simulink library "Generator_Lib"  (R2014a)
settings: Solver=ode45  StartTime=0.0  StopTime=10.0  RelTol=1e-3
undefined symbols (not defined in the file): block_angle, D1, Delta, DiscIntNeverNeededParam, fao, gcbh, sps_rtmsupport, Ts
libraries: powerlib x73, simulink x16, powerlib_extras x13, Generator_Lib x3, sps_avr x2, powerlib_meascontrol x2, spsSimpleSynchronousMachineModel x2
(part 1 of 3)
Description:
  | Copyright 2014 The MathWorks, Inc.
settings Model: Creator=smiller  LastModifiedBy=psanghvi

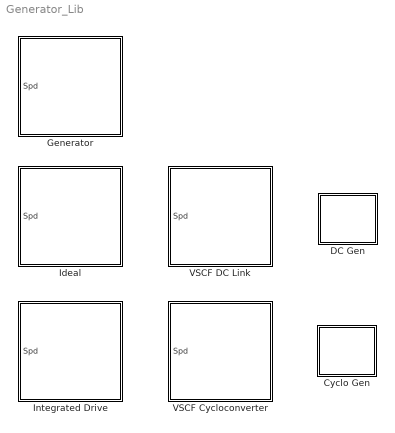
== system Generator_Lib ==
  Cyclo Gen : Subsystem
  DC Gen : Subsystem
  Generator : Subsystem  BlockChoice=Integrated Drive
      settings: TemplateBlock=self  MemberBlocks=Ideal,Integrated Drive,VSCF Cycloconverter,VSCF DC Link
  Ideal : Subsystem
      mask Display:
      | image(imread('Gen_Ideal_IMAGE.JPG','jpg'))
      | %port_label('RConn',1,'A');
      | %port_label('RConn',2,'B');
      | %port_label('RConn',3,'C');
      | %port_label('Input',1,'Spd');
  Integrated Drive : Subsystem
      mask Display:
      | image(imread('Gen_IDG_IMAGE.JPG','jpg'))
      | %port_label('RConn',1,'A');
      | %port_label('RConn',2,'B');
      | %port_label('RConn',3,'C');
      | %port_label('Input',1,'Spd');
  VSCF Cycloconverter : Subsystem
      mask Display:
      | image(imread('Gen_VSCF_Cycloconverter_IMAGE.JPG','jpg'))
      | %port_label('RConn',1,'A');
      | %port_label('RConn',2,'B');
      | %port_label('RConn',3,'C');
      | %port_label('Input',1,'Spd');
  VSCF DC Link : Subsystem
      mask Display:
      | image(imread('Gen_VSCF_DCLink_IMAGE.JPG','jpg'))
      | %port_label('RConn',1,'A');
      | %port_label('RConn',2,'B');
      | %port_label('RConn',3,'C');
      | %port_label('Input',1,'Spd');

== system Generator_Lib/Cyclo Gen ==
  Ideal : Subsystem
      mask Display:
      | image(imread('Gen_Ideal_Var_IMAGE.jpg'));
      | port_label('RConn',1,'A');
      | port_label('RConn',2,'B');
      | port_label('RConn',3,'C');
      | port_label('Input',1,'rpm');

== system Generator_Lib/DC Gen ==
  DC Link Gen : Subsystem  BlockChoice=Ideal
      settings: TemplateBlock=self  MemberBlocks=Ideal,Sync Mach
  Ideal : Subsystem
      mask Display: image(imread('Gen_Ideal_Var_IMAGE.jpg'));
  Sync Mach : Subsystem
      mask Display: image(imread('Gen_Sync_Machine_IMAGE.jpg'));

== system Generator_Lib/Generator ==
  Spd : Inport
  Integrated Drive : Generator_Lib/Integrated Drive  SystemSampleTime=-1
  A : PMIOPort  Port=1  Side=Right
  B : PMIOPort  Port=2  Side=Right
  C : PMIOPort  Port=3  Side=Right
  wires:
  Spd/1 -> Integrated Drive/1
  connections:
  Integrated Drive/RConn1 -- A/RConn1
  Integrated Drive/RConn2 -- B/RConn1
  Integrated Drive/RConn3 -- C/RConn1

== system Generator_Lib/Ideal ==
  Spd : Inport
  Parasitic Resistive Load : powerlib/Elements/Three-Phase Series RLC Load  LConnTagsString=A|B|C  Configuration=Y (grounded)  NominalVoltage=200  NominalFrequency=400  ActivePower=5000  InductivePower=0  CapacitivePower=0  Measurements=None  LoadType=constant Z
  Sensing : Subsystem
      mask Display: disp('S')
  Terminator : Terminator
  Three-Phase V-I Measurement4 : powerlib/Measurements/Three-Phase V-I Measurement  VoltageMeasurement=phase-to-ground  SetLabelV=on  LabelV=Vabc_Gen1Only  Vpu=off  VpuLL=off  CurrentMeasurement=yes  SetLabelI=on  LabelI=Iabc_Gen1Only  Ipu=off  Pbase=100e6  Vbase=500e3  OutputType=Magnitude  PhasorSimulation=on  PSBequivalent=0
  Three-Phase Source : powerlib/Electrical Sources/Three-Phase Source  Voltage=200  PhaseAngle=0  Frequency=400  InternalConnection=Yg  SpecifyImpedance=off  Resistance=0.1*0  Inductance=0.01*0  ShortCircuitLevel=0.1  BaseVoltage=200  XRratio=7  BusType=swing  Pref=0  Qref=0  Qmin=-inf  Qmax=inf
  Vab : Subsystem
  rpm2 radps : Gain  Gain=pi/30
  A : PMIOPort  Port=1  Side=Right
  B : PMIOPort  Port=2  Side=Right
  C : PMIOPort  Port=3  Side=Right
  wires:
  Spd/1 -> rpm2 radps/1
  rpm2 radps/1 -> Terminator/1
  connections:
  Vab/RConn2 -- Three-Phase V-I Measurement4/RConn2 -- Parasitic Resistive Load/LConn2 -- B/RConn1
  Parasitic Resistive Load/LConn3 -- Three-Phase V-I Measurement4/RConn3 -- C/RConn1
  Vab/RConn1 -- Three-Phase V-I Measurement4/RConn1 -- Parasitic Resistive Load/LConn1 -- A/RConn1
  Three-Phase V-I Measurement4/LConn1 -- Three-Phase Source/RConn1
  Three-Phase V-I Measurement4/LConn2 -- Three-Phase Source/RConn2
  Three-Phase V-I Measurement4/LConn3 -- Three-Phase Source/RConn3

== system Generator_Lib/Integrated Drive ==
  Spd : Inport
  Bus Selector2 : BusSelector  OutputSignals=Rotor speed wm (rad/s)
  Displays : Subsystem
  Generator Control Unit (GCU) : Subsystem
      mask Display: %image(imread('power_aircraft_distribution_GCU.jpg','jpg'))
  Generator Control Breaker (GCB) : Subsystem
  IDG : Subsystem
  Parasitic Resistive Load : powerlib/Elements/Three-Phase Series RLC Load  LConnTagsString=A|B|C  Configuration=Y (grounded)  NominalVoltage=200  NominalFrequency=400  ActivePower=5000  InductivePower=0  CapacitivePower=0  Measurements=None  LoadType=constant Z
  Sensing : Subsystem
      mask Display: disp('S')
  Simplified Synchronous Machine SI Units : powerlib/Machines/Simplified Synchronous Machine SI Units  ConnectionType=3-wire Y  MechanicalLoad=Speed w  MeasurementBus=off  NominalParameters=[50e3 200 400]  Mechanical=[0.02 0 2]  InternalRL="[0.0204  0.08104e-3]"  InitialConditions=[-99 1.73677 24.5109 24.5109 24.5109 -1.98949 -121.989 118.011]  Units=1  LoadFlowParameters=[1 0 0 0 0]  TsPowergui=0  TsBlock=-1  BusType=swing  Pref=0  Qref=0  Qmin=-inf  Qmax=+inf  PLF=0  QLF=0
  Vab : Subsystem
  A : PMIOPort  Port=1  Side=Right
  B : PMIOPort  Port=2  Side=Right
  C : PMIOPort  Port=3  Side=Right
  wires:
  Simplified Synchronous Machine SI Units/1 -> Sensing/1(In1), Bus Selector2/1
  Generator Control Breaker (GCB)/1(Vabc) -> Generator Control Unit (GCU)/2(Vabc)
  Bus Selector2/1 -> Generator Control Breaker (GCB)/1(GLC), Generator Control Unit (GCU)/3(PMG), Displays/1(w)  "<Rotor speed wm (rad/s)>"
  Generator Control Unit (GCU)/1(V Field) -> Simplified Synchronous Machine SI Units/2  "Field"
  Generator Control Breaker (GCB)/2(Iabc) -> Generator Control Unit (GCU)/1(Iabc)
  Spd/1 -> IDG/1(Tur)
  IDG/1(Dr) -> Simplified Synchronous Machine SI Units/1
  connections:
  A/RConn1 -- Vab/RConn1 -- Generator Control Breaker (GCB)/RConn1
  C/RConn1 -- Generator Control Breaker (GCB)/RConn3
  B/RConn1 -- Vab/RConn2 -- Generator Control Breaker (GCB)/RConn2
  Generator Control Breaker (GCB)/LConn3 -- Parasitic Resistive Load/LConn3 -- Simplified Synchronous Machine SI Units/RConn3
  Parasitic Resistive Load/LConn2 -- Generator Control Breaker (GCB)/LConn2 -- Simplified Synchronous Machine SI Units/RConn2
  Parasitic Resistive Load/LConn1 -- Generator Control Breaker (GCB)/LConn1 -- Simplified Synchronous Machine SI Units/RConn1

== system Generator_Lib/VSCF Cycloconverter ==
  Spd : Inport
  AC Generator Cycloconverter : Subsystem
  Constant : Constant  Value=[0 0 0]
  Generator Control Breaker (GCB) : Subsystem
  Terminator : Terminator
  Terminator1 : Terminator
  Vab : Subsystem
  A : PMIOPort  Port=1  Side=Right
  B : PMIOPort  Port=2  Side=Right
  C : PMIOPort  Port=3  Side=Right
  tag scope: Gen1Bus=global
  wires:
  Spd/1 -> AC Generator Cycloconverter/1(rpm), Generator Control Breaker (GCB)/1(GLC)
  Constant/1 -> [Gen1Bus]
  Generator Control Breaker (GCB)/1(Vabc) -> Terminator/1
  Generator Control Breaker (GCB)/2(Iabc) -> Terminator1/1
  connections:
  Vab/RConn1 -- Generator Control Breaker (GCB)/RConn1 -- A/RConn1
  C/RConn1 -- Generator Control Breaker (GCB)/RConn3
  Vab/RConn2 -- Generator Control Breaker (GCB)/RConn2 -- B/RConn1
  AC Generator Cycloconverter/RConn3 -- Generator Control Breaker (GCB)/LConn3
  AC Generator Cycloconverter/RConn2 -- Generator Control Breaker (GCB)/LConn2
  AC Generator Cycloconverter/RConn1 -- Generator Control Breaker (GCB)/LConn1

== system Generator_Lib/VSCF DC Link ==
  note: AC-DC-AC PWM Converter
  Spd : Inport
  Constant : Constant  Value=[0 0 0]
  DC Link Gen : Subsystem  BlockChoice=Ideal
      settings: AttributesFormatString=%<BlockChoice>  TemplateBlock=Generator_Lib/DC Gen/DC Link Gen  MemberBlocks=Ideal,Sync Mach
  LC Filter : Subsystem
  Meas : powerlib/Measurements/Three-Phase V-I Measurement  VoltageMeasurement=phase-to-ground  SetLabelV=off  LabelV=V1  Vpu=on  VpuLL=off  CurrentMeasurement=no  SetLabelI=off  LabelI=I1  Ipu=off  Pbase=1e3  Vbase=200  OutputType=Magnitude  PhasorSimulation=off  PSBequivalent=0
  Rect and Inv : Subsystem
  Regulator : Subsystem
  Subsystem2 : Subsystem
      mask Display: disp('S')
  Subsystem4 : Subsystem
      mask Display: disp('S')
  Subsystem5 : Subsystem
      mask Display: disp('S')
  Transformer : powerlib/Elements/Three-Phase Transformer (Two Windings)  Winding1Connection=Yg  UNITS=pu  NominalPower=[ 50e3 , 800 ]  Winding1=[ 200 , 0.004 , 0.02 ]  Winding2Connection=Delta (D1)  Winding2=[ 600 , 0.004 , 0.02 ]  SetSaturation=off  Rm=200  Lm=200  Saturation="[ 0,0  ;  0.005,1.2  ;  1.0,1.4 ]"  Hysteresis=off  DataFile='hysteresis'  SetInitialFlux=off  InitialFluxes=[ 0.8 , -0.8 , 0.7 ]  Measurements=None  MoreParameters=off  BreakLoop=off  DataType=off  TransfoNumber=0
  "Vref (pu) " : Constant
  A : PMIOPort  Port=1  Side=Right
  B : PMIOPort  Port=2  Side=Right
  C : PMIOPort  Port=3  Side=Right
  tag scope: Gen1Bus=global
  wires:
  "Vref (pu) "/1 -> Regulator/1(Vref (pu))
  Meas/1 -> Regulator/2(Vabc (pu))
  Regulator/1(g) -> Rect and Inv/1(g)
  Spd/1 -> DC Link Gen/1(rpm)
  Constant/1 -> [Gen1Bus]
  connections:
  Subsystem4/LConn1 -- A/RConn1 -- Meas/RConn1
  Transformer/LConn1 -- DC Link Gen/RConn1 -- Subsystem2/LConn1
  LC Filter/LConn2 -- Rect and Inv/RConn2 -- Subsystem5/LConn2
  LC Filter/LConn1 -- Subsystem5/LConn1 -- Rect and Inv/RConn1
  B/RConn1 -- Meas/RConn2
  Meas/LConn1 -- LC Filter/RConn1
  DC Link Gen/RConn2 -- Transformer/LConn2
  Meas/LConn2 -- LC Filter/RConn2
  Meas/RConn3 -- C/RConn1
  Meas/LConn3 -- LC Filter/RConn3
  Transformer/RConn1 -- Rect and Inv/LConn1
  DC Link Gen/RConn3 -- Transformer/LConn3
  Rect and Inv/LConn2 -- Transformer/RConn2
  Transformer/RConn3 -- Rect and Inv/LConn3
  Rect and Inv/RConn3 -- LC Filter/LConn3

== system Generator_Lib/Cyclo Gen/Ideal ==
  rpm : Inport
  Cycloconverter control (Vsync) : Subsystem
  Ground1 : powerlib/Elements/Ground  LConnTagsString=a
  Ideal Source : Subsystem
  Load Measurements : powerlib/Measurements/Three-Phase V-I Measurement  VoltageMeasurement=phase-to-ground  SetLabelV=on  LabelV=Vload  Vpu=off  VpuLL=off  CurrentMeasurement=yes  SetLabelI=on  LabelI=Iload  Ipu=off  Pbase=100e6  Vbase=500e3  OutputType=Complex  PhasorSimulation=off  PSBequivalent=0
  Phase A Cycloconverter : Subsystem
  Phase B Cycloconverter : Subsystem
  Phase C Cycloconverter : Subsystem
  Source Measurements : powerlib/Measurements/Three-Phase V-I Measurement  VoltageMeasurement=phase-to-ground  SetLabelV=on  LabelV=Vsource  Vpu=off  VpuLL=off  CurrentMeasurement=yes  SetLabelI=on  LabelI=Isource  Ipu=off  Pbase=100e6  Vbase=500e3  OutputType=Complex  PhasorSimulation=off  PSBequivalent=0
  Three-Phase Transformer (Two Windings)1 : powerlib/Elements/Three-Phase Transformer (Two Windings)  Winding1Connection=Delta (D1)  UNITS=pu  NominalPower=[3e6 3000]  Winding1=[200 0 0]  Winding2Connection=Delta (D1)  Winding2=[200/sqrt(3) 1e-8 0]  SetSaturation=off  Rm=Inf  Lm=Inf  Saturation=[ 0,0 ; 0.0024,1.2 ; 1.0,1.52 ]  Hysteresis=off  DataFile='hysteresis'  SetInitialFlux=off  InitialFluxes=[ 0.8 , -0.8 , 0.7 ]  Measurements=None  MoreParameters=off  BreakLoop=off  DataType=off  TransfoNumber=1
  Three-Phase Transformer (Two Windings)2 : powerlib/Elements/Three-Phase Transformer (Two Windings)  Winding1Connection=Delta (D1)  UNITS=pu  NominalPower=[3e6 3000]  Winding1=[200 0 0]  Winding2Connection=Delta (D1)  Winding2=[200/sqrt(3) 1e-8 0]  SetSaturation=off  Rm=Inf  Lm=Inf  Saturation=[ 0,0 ; 0.0024,1.2 ; 1.0,1.52 ]  Hysteresis=off  DataFile='hysteresis'  SetInitialFlux=off  InitialFluxes=[ 0.8 , -0.8 , 0.7 ]  Measurements=None  MoreParameters=off  BreakLoop=off  DataType=off  TransfoNumber=1
  Three-Phase Transformer (Two Windings)3 : powerlib/Elements/Three-Phase Transformer (Two Windings)  Winding1Connection=Delta (D1)  UNITS=pu  NominalPower=[3e6 3000]  Winding1=[200 0 0]  Winding2Connection=Delta (D1)  Winding2=[200/sqrt(3) 1e-8 0]  SetSaturation=off  Rm=Inf  Lm=Inf  Saturation=[ 0,0 ; 0.0024,1.2 ; 1.0,1.52 ]  Hysteresis=off  DataFile='hysteresis'  SetInitialFlux=off  InitialFluxes=[ 0.8 , -0.8 , 0.7 ]  Measurements=None  MoreParameters=off  BreakLoop=off  DataType=off  TransfoNumber=1
  Vsync Measurement : powerlib/Measurements/Three-Phase V-I Measurement  VoltageMeasurement=phase-to-phase  SetLabelV=on  LabelV=Vsync  Vpu=off  VpuLL=off  CurrentMeasurement=no  SetLabelI=off  LabelI=Iabc  Ipu=off  Pbase=100e6  Vbase=500e3  OutputType=Complex  PhasorSimulation=off  PSBequivalent=0
  A : PMIOPort  Port=1  Side=Right
  B : PMIOPort  Port=2  Side=Right
  C : PMIOPort  Port=3  Side=Right
  wires:
  rpm/1 -> Ideal Source/1(rpm)
  connections:
  Load Measurements/RConn1 -- A/RConn1
  Phase A Cycloconverter/LConn2 -- Vsync Measurement/RConn2
  Three-Phase Transformer (Two Windings)3/RConn3 -- Vsync Measurement/LConn3
  Phase C Cycloconverter/RConn2 -- Phase A Cycloconverter/RConn2 -- Phase B Cycloconverter/RConn2 -- Ground1/LConn1
  Three-Phase Transformer (Two Windings)2/RConn2 -- Phase C Cycloconverter/LConn2
  Source Measurements/RConn3 -- Three-Phase Transformer (Two Windings)3/LConn3 -- Three-Phase Transformer (Two Windings)2/LConn3 -- Three-Phase Transformer (Two Windings)1/LConn3
  Phase B Cycloconverter/RConn1 -- Load Measurements/LConn2
  Vsync Measurement/RConn1 -- Phase A Cycloconverter/LConn1
  Phase B Cycloconverter/LConn1 -- Three-Phase Transformer (Two Windings)1/RConn1
  Phase B Cycloconverter/LConn2 -- Three-Phase Transformer (Two Windings)1/RConn2
  Three-Phase Transformer (Two Windings)3/RConn1 -- Vsync Measurement/LConn1
  Phase C Cycloconverter/LConn1 -- Three-Phase Transformer (Two Windings)2/RConn1
  Phase A Cycloconverter/RConn1 -- Load Measurements/LConn1
  Source Measurements/RConn1 -- Three-Phase Transformer (Two Windings)3/LConn1 -- Three-Phase Transformer (Two Windings)2/LConn1 -- Three-Phase Transformer (Two Windings)1/LConn1
  Source Measurements/RConn2 -- Three-Phase Transformer (Two Windings)3/LConn2 -- Three-Phase Transformer (Two Windings)2/LConn2 -- Three-Phase Transformer (Two Windings)1/LConn2
  Phase C Cycloconverter/RConn1 -- Load Measurements/LConn3
  Vsync Measurement/RConn3 -- Phase A Cycloconverter/LConn3
  Load Measurements/RConn3 -- C/RConn1
  Phase C Cycloconverter/LConn3 -- Three-Phase Transformer (Two Windings)2/RConn3
  Source Measurements/LConn2 -- Ideal Source/RConn2
  Three-Phase Transformer (Two Windings)3/RConn2 -- Vsync Measurement/LConn2
  Ideal Source/RConn1 -- Source Measurements/LConn1
  Load Measurements/RConn2 -- B/RConn1
  Ideal Source/RConn3 -- Source Measurements/LConn3
  Three-Phase Transformer (Two Windings)1/RConn3 -- Phase B Cycloconverter/LConn3

== system Generator_Lib/DC Gen/DC Link Gen ==
  rpm : Inport
  Ideal : Generator_Lib/DC Gen/Ideal  SystemSampleTime=-1
  A : PMIOPort  Port=1  Side=Right
  B : PMIOPort  Port=2  Side=Right
  C : PMIOPort  Port=3  Side=Right
  wires:
  rpm/1 -> Ideal/1
  connections:
  Ideal/RConn1 -- A/RConn1
  Ideal/RConn2 -- B/RConn1
  Ideal/RConn3 -- C/RConn1

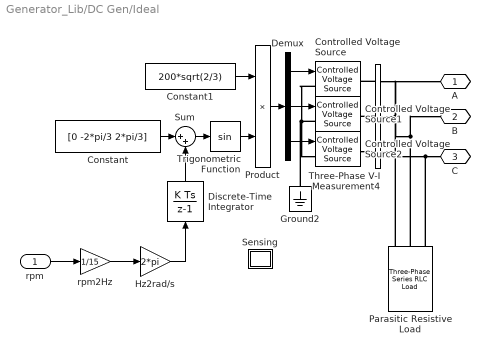
== system Generator_Lib/DC Gen/Ideal ==
  rpm : Inport
  Constant : Constant  Value=[0 -2*pi/3 2*pi/3]
  Constant1 : Constant  Value=200*sqrt(2/3)
  Controlled Voltage Source : powerlib/Electrical Sources/Controlled Voltage Source  Initialize=off  Source_Type=AC  Amplitude=0  Phase=0  Frequency=0  Measurements=None
  Controlled Voltage Source1 : powerlib/Electrical Sources/Controlled Voltage Source  Initialize=off  Source_Type=AC  Amplitude=0  Phase=0  Frequency=0  Measurements=None
  Controlled Voltage Source2 : powerlib/Electrical Sources/Controlled Voltage Source  Initialize=off  Source_Type=AC  Amplitude=0  Phase=0  Frequency=0  Measurements=None
  Demux : Demux  Outputs=3
  Discrete-Time Integrator : DiscreteIntegrator  SampleTime=Ts  ICPrevOutput=DiscIntNeverNeededParam  ICPrevScaledInput=DiscIntNeverNeededParam
  Ground2 : powerlib/Elements/Ground  LConnTagsString=a
  Hz2rad/s : Gain  Gain=2*pi
  Parasitic Resistive Load : powerlib/Elements/Three-Phase Series RLC Load  LConnTagsString=A|B|C  Configuration=Y (grounded)  NominalVoltage=200  NominalFrequency=400  ActivePower=5000  InductivePower=0  CapacitivePower=0  Measurements=None  LoadType=constant Z
  Product : Product
  Sensing : Subsystem
      mask Display: disp('S')
  Sum : Sum  Inputs=|++
  Three-Phase V-I Measurement4 : powerlib/Measurements/Three-Phase V-I Measurement  VoltageMeasurement=phase-to-ground  SetLabelV=on  LabelV=Vabc_Gen1Only  Vpu=off  VpuLL=off  CurrentMeasurement=yes  SetLabelI=on  LabelI=Iabc_Gen1Only  Ipu=off  Pbase=100e6  Vbase=500e3  OutputType=Magnitude  PhasorSimulation=on  PSBequivalent=0
  Trigonometric Function : Trigonometry
  rpm2Hz : Gain  Gain=1/15
  A : PMIOPort  Port=1  Side=Right
  B : PMIOPort  Port=2  Side=Right
  C : PMIOPort  Port=3  Side=Right
  wires:
  rpm/1 -> rpm2Hz/1
  Discrete-Time Integrator/1 -> Sum/2
  Constant1/1 -> Product/1
  Constant/1 -> Sum/1
  Hz2rad/s/1 -> Discrete-Time Integrator/1
  Sum/1 -> Trigonometric Function/1
  Trigonometric Function/1 -> Product/2
  Product/1 -> Demux/1
  Demux/1 -> Controlled Voltage Source/1
  Demux/2 -> Controlled Voltage Source1/1
  Demux/3 -> Controlled Voltage Source2/1
  rpm2Hz/1 -> Hz2rad/s/1
  connections:
  Controlled Voltage Source/LConn1 -- Ground2/LConn1 -- Controlled Voltage Source2/LConn1 -- Controlled Voltage Source1/LConn1
  Three-Phase V-I Measurement4/LConn1 -- Controlled Voltage Source/RConn1
  Three-Phase V-I Measurement4/LConn2 -- Controlled Voltage Source1/RConn1
  Controlled Voltage Source2/RConn1 -- Three-Phase V-I Measurement4/LConn3
  Three-Phase V-I Measurement4/RConn3 -- Parasitic Resistive Load/LConn3 -- C/RConn1
  Three-Phase V-I Measurement4/RConn2 -- Parasitic Resistive Load/LConn2 -- B/RConn1
  Three-Phase V-I Measurement4/RConn1 -- A/RConn1 -- Parasitic Resistive Load/LConn1

== system Generator_Lib/DC Gen/Sync Mach ==
  rpm : Inport
  Bus Selector2 : BusSelector  OutputSignals=Rotor speed wm (rad/s)
  Displays : Subsystem
  Generator Control Unit (GCU) : Subsystem
      mask Display: %image(imread('power_aircraft_distribution_GCU.jpg','jpg'))
  Generator Control Breaker (GCB) : Subsystem
  Parasitic Resistive Load : PMComponent  DialogController=POWERSYS.PowerSysDialog  LoadFcn=sps_rtmsupport('LoadFcn',gcbh);  StartFcn=sps_rtmsupport('StartFcn',gcbh);  StopFcn=sps_rtmsupport('StopFcn',gcbh);  PhysicalDomain=powersysdomain  LeftPortType=p1  RightPortType=p1  LConnTagsString=A|B|C  mask(Three-Phase Series RLC Load){Configuration=Y (grounded), NominalVoltage=200, NominalFrequency=800, ActivePower=5000, InductivePower=0, CapacitivePower=0, Measurements=None, LoadType=constant Z}
      mask prompts: NominalVoltage "Nominal phase-to-phase voltage Vn (Vrms)"; NominalFrequency "Nominal frequency fn (Hz):"; ActivePower "Active power P (W):"; InductivePower "Inductive reactive power QL (positive var):"; CapacitivePower "Capacitive reactive power Qc (negative var):"; LoadType "Load type"
      mask help: Implements a three-phase series RLC load.
      mask init:
      | [s1,s2,s3,s4,r1,r2,l1,l2,c1,c2,c3,c4] = powericon('Series RLC Load',ActivePower,InductivePower,CapacitivePower);
      | ground = Configuration==1;
      | neutral = Configuration==3;
      | power_initmask();
      settings: AttributesFormatString=\n  CopyFcn=sps_rtmsupport('CopyFcn',gcbh);  DeleteFcn=sps_rtmsupport('DeleteFcn',gcbh);  UndoDeleteFcn=sps_rtmsupport('UndoDeleteFcn',gcbh);  ModelCloseFcn=sps_rtmsupport('ModelCloseFcn',gcbh);  PreSaveFcn=sps_rtmsupport('PreSaveFcn',gcbh);  PostSaveFcn=sps_rtmsupport('PostSaveFcn',gcbh);  NameChangeFcn=sps_rtmsupport('NameChangeFcn',gcbh);  PreCopyFcn=sps_rtmsupport('PreCopyFcn',gcbh);  OpenFcn=sps_rtmsupport('OpenFcn',gcbh, [1 7 8]);  CloseFcn=sps_rtmsupport('CloseFcn',gcbh);  PreDeleteFcn=sps_rtmsupport('PreDeleteFcn',gcbh);
      mask Help: helpview(psbhelp);
      mask TypeOptions Configuration: Y (grounded) | Y (floating) | Y (neutral) | Delta
      mask Callback Configuration: powericon('psbcallbacks',gcb,'Three-Phase Series RLC Load');
      mask TypeOptions Measurements: None | Branch voltages | Branch currents | Branch voltages and currents
      mask TypeOptions LoadType: constant Z | constant PQ
      mask Display:
      | plot(s1-60,s2,s3+80,s4,r1,r2,l1,l2,c1,c2,c3,c4)
      | 
      | plot( ground*[s3,s3], ground*[-s2/4,s2/4])
      | plot( ground*[s3+30,s3+30], ground*[-s2/6,s2/6])
      | plot( ground*[s3+60,s3+60], ground*[-s2/10,s2/10])
      | 
      | plot( neutral*[s3,s3+80], neutral*[0,0])
      | 
      | port_label('LConn', 1, 'A')
      | port_label('LConn', 2, 'B')
      | port_label('LConn', 3, 'C')
  Sensing : Subsystem
      mask Display: disp('S')
  Simplified Synchronous Machine SI Units : Subsystem  DialogController=POWERSYS.PowerSysDialog  LoadFcn=sps_rtmsupport('LoadFcn',gcbh);  StartFcn=sps_rtmsupport('StartFcn',gcbh);  StopFcn=sps_rtmsupport('StopFcn',gcbh);  mask(Simplified Synchronous Machine){ConnectionType=3-wire Y, MechanicalLoad=Speed w, NominalParameters=[50e3 200 800], Mechanical=[0.02 0 2*2], InternalRL=[0.0204  0.08104e-3], InitialConditions=[-99 1.73677 24.5109 24.5109 24.5109 -1.98949 -121.989 118.011], Units=1, LoadFlowParameters=[1 0 0 0 0], TsPowergui=0, TsBlock=-1, BusType=swing, Pref=0, Qref=0, Qmin=-inf, Qmax=+inf, PLF=0, QLF=0}
      mask prompts: ConnectionType "Connection type:"; MechanicalLoad "Mechanical input:"; NominalParameters "Nominal power, line-to-line voltage, and frequency [ Pn(VA) Vn(Vrms) fn(Hz) ]:"; Mechanical "Inertia, damping factor and pairs of poles [J(kg.m^2) Kd(pu_T/pu_w) p()]"; InternalRL "Internal impedance [ R(ohm)  L(H) ]:"; InitialConditions "Initial conditions [ dw(%)  th(deg)  ia,ib,ic(A)  pha,phb,phc(deg) ]:"; Units "iounits"; LoadFlowParameters "Load Flow Parameters"; TsPowergui "Sample time of powergui block"; TsBlock "Sample time (-1 for inherited)"; BusType "Generation type"; Pref "Active power generation P (W)"; Qref "Reactive power generation Q (var)"; Qmin "Minimum reactive power Qmin (var)"; Qmax "Maximum reactive power Qmax (var)"; PLF "Load flow solution P_LF (W)"; QLF "Load flow solution Q_LF (var)"
      mask help:
      | Implements a 3-phase simplified synchronous machine. Machine is modelled as an internal voltage behind a R-L impedance. Stator windings are connected in wye to an internal neutral point.
      |
      | Use this block if you want to specify SI  parameters.
      mask init:
      | block = gcb;
      | [Ts,SSM,WantBlockChoice,X,Y] = powericon('SimplifiedSynchronousMachineInit',block,TsPowergui,TsBlock,MechanicalLoad,'SI',ConnectionType,NominalParameters,Mechanical,InternalRL,InitialConditions,0,-1);
      | powericon('SetInternalModels','set',block,WantBlockChoice);
      | powericon('ShaftInput',block);
      settings: CopyFcn=sps_rtmsupport('CopyFcn',gcbh); powericon('psbloadfunction',gcb,'gotofrom','UpdateGotoTag');  DeleteFcn=sps_rtmsupport('DeleteFcn',gcbh);  UndoDeleteFcn=sps_rtmsupport('UndoDeleteFcn',gcbh);  ModelCloseFcn=sps_rtmsupport('ModelCloseFcn',gcbh);  PreSaveFcn=sps_rtmsupport('PreSaveFcn',gcbh);  PostSaveFcn=sps_rtmsupport('PostSaveFcn',gcbh);  NameChangeFcn=sps_rtmsupport('NameChangeFcn',gcbh);  PreCopyFcn=sps_rtmsupport('PreCopyFcn',gcbh);  OpenFcn=sps_rtmsupport('OpenFcn',gcbh, [1 2 11]);  CloseFcn=sps_rtmsupport('CloseFcn',gcbh);  PreDeleteFcn=sps_rtmsupport('PreDeleteFcn',gcbh);
      mask Help: helpview(psbhelp);
      mask TypeOptions ConnectionType: 3-wire Y | 4-wire Y
      mask Callback ConnectionType: powericon('SimplifiedSynchronousMachineCback',gcb);
      mask TypeOptions MechanicalLoad: Mechanical power Pm | Speed w | Mechanical rotational port
      mask TypeOptions BusType: swing | PV | PQ
      mask Callback BusType: powericon('SimplifiedSynchronousMachineCback',gcb);
      mask Display:
      | plot(X.p1,Y.p1,X.p2,Y.p2,X.p3,Y.p3,X.p4,Y.p4,X.p5,Y.p5,X.p6,Y.p6,X.p7,Y.p7);
      | disp('\nSSM');
      | color('blue');
      | plot(X.p8,Y.p8);
      | plot(X.p9,Y.p9);
      | plot(X.p10,Y.p10);
      | plot(X.p11,Y.p11);
      | port_label('input',1,SSM.PortLabel)
  Vab : Subsystem
  rpm2 radps : Gain  Gain=pi/30
  A : PMIOPort  Port=1  Side=Right
  B : PMIOPort  Port=2  Side=Right
  C : PMIOPort  Port=3  Side=Right
  wires:
  rpm/1 -> rpm2 radps/1
  Generator Control Breaker (GCB)/2(Iabc) -> Generator Control Unit (GCU)/1(Iabc)
  Generator Control Unit (GCU)/1(V Field) -> Simplified Synchronous Machine SI Units/2(E)  "Field"
  Bus Selector2/1 -> Generator Control Breaker (GCB)/1(GLC), Generator Control Unit (GCU)/3(PMG), Displays/1(w)  "<Rotor speed wm (rad/s)>"
  Generator Control Breaker (GCB)/1(Vabc) -> Generator Control Unit (GCU)/2(Vabc)
  rpm2 radps/1 -> Simplified Synchronous Machine SI Units/1(mec)
  Simplified Synchronous Machine SI Units/1(m) -> Sensing/1(In1), Bus Selector2/1
  connections:
  C/RConn1 -- Generator Control Breaker (GCB)/RConn3
  Generator Control Breaker (GCB)/LConn1 -- Simplified Synchronous Machine SI Units/RConn1 -- Parasitic Resistive Load/LConn1
  Generator Control Breaker (GCB)/LConn2 -- Simplified Synchronous Machine SI Units/RConn2 -- Parasitic Resistive Load/LConn2
  Parasitic Resistive Load/LConn3 -- Simplified Synchronous Machine SI Units/RConn3 -- Generator Control Breaker (GCB)/LConn3
  Generator Control Breaker (GCB)/RConn2 -- B/RConn1 -- Vab/RConn2
  Generator Control Breaker (GCB)/RConn1 -- A/RConn1 -- Vab/RConn1

== system Generator_Lib/Ideal/Sensing ==
  Constant : Constant  Value=[1 1]*12000  SampleTime=-1
  Constant1 : Constant  Value=202  SampleTime=-1
  Mux : Mux  Inputs=3
  rpm2pu1 : Gain  Gain=2*pi/60
  tag scope: Gen1Data=global
  wires:
  [Pwr_Gen1_Only] -> Mux/3
  Constant1/1 -> Mux/2
  rpm2pu1/1 -> Mux/1
  Mux/1 -> [Gen1Data]
  Constant/1 -> rpm2pu1/1  "Spd"

== system Generator_Lib/Ideal/Vab ==
  Voltage Measurement : powerlib/Measurements/Voltage Measurement  PhasorSimulation=off  OutputType=Magnitude  PSBequivalent=0
  + : PMIOPort  Port=1  Side=Right
  - : PMIOPort  Port=2  Side=Right
  tag scope: Gen1_Vab=global
  wires:
  Voltage Measurement/1 -> [Gen1_Vab]
  connections:
  Voltage Measurement/LConn1 -- +/RConn1
  Voltage Measurement/LConn2 -- -/RConn1

== system Generator_Lib/Integrated Drive/Displays ==
  w : Inport
  Frequency (Hz) : Display
      settings: Decimation=100  SampleTime=1e-2
  Gain : Gain  Gain=30/pi
  Gain3 : Gain  Gain=1/30
  Rate Transition : RateTransition  OutPortSampleTimeOpt=Inherit  OutPortSampleTime=Ts
  Rate Transition1 : RateTransition  OutPortSampleTimeOpt=Inherit  OutPortSampleTime=Ts
  Speed (RPM) : Display
      settings: Decimation=100  SampleTime=1e-2
  wires:
  w/1 -> Gain/1
  Rate Transition/1 -> Speed (RPM)/1
  Gain3/1 -> Rate Transition1/1
  Gain/1 -> Rate Transition/1, Gain3/1
  Rate Transition1/1 -> Frequency (Hz)/1

== system Generator_Lib/Integrated Drive/Generator Control Unit (GCU) ==
  Iabc : Inport
  Vabc : Inport  Port=2
  PMG : Inport  Port=3
  Demux : Demux  Outputs=3
  Excitation System : sps_avr/Excitation System  tr=20e-3  reg=[ 300, 0.001 ]  exc=[ 1, 0 ]  tgr=[ 0, 0 ]  damp=[ 0.001, 0.1 ]  sat=[ 0, 0 ]  lim=[ -2, 2, 0 ]  v0=[1 1*203.1/200]
  Integrator : Integrator
  PU_SI : Gain  Gain=200
  SI_PU : Gain  Gain=1/(200*sqrt(2))
  Terminator1 : Terminator
  Terminator2 : Terminator
  Vref : Constant
  abc to dq0 : powerlib_meascontrol/Transformations/abc to dq0  Alignment=90 degrees behind phase A axis
  threshold3 : Constant  Value=0
  V Field : Outport
  tag scope: Gen1_Vfield=global
  wires:
  Vabc/1 -> SI_PU/1
  PMG/1 -> Integrator/1
  Integrator/1 -> abc to dq0/2
  abc to dq0/1 -> Demux/1
  Demux/1 -> Excitation System/2
  Demux/2 -> Excitation System/3
  SI_PU/1 -> abc to dq0/1
  Excitation System/1 -> PU_SI/1
  PU_SI/1 -> V Field/1, [Gen1_Vfield]
  Vref/1 -> Excitation System/1
  threshold3/1 -> Excitation System/4
  Iabc/1 -> Terminator1/1
  Demux/3 -> Terminator2/1

== system Generator_Lib/Integrated Drive/Generator Control Breaker (GCB) ==
  GLC : Inport
  Close switch : Subsystem
  Complex to Real-Imag : ComplexToRealImag  Output=Real
  Complex to Real-Imag1 : ComplexToRealImag  Output=Real
  Contactor : Subsystem
  Memory : Memory
  P.O.R  and CTA : powerlib/Measurements/Three-Phase V-I Measurement  VoltageMeasurement=phase-to-phase  SetLabelV=off  LabelV=Vabc_Gen1  Vpu=off  VpuLL=off  CurrentMeasurement=yes  SetLabelI=off  LabelI=Iabc_Gen1  Ipu=off  Pbase=100e6  Vbase=500e3  OutputType=Complex  PhasorSimulation=off  PSBequivalent=0
  in_a : PMIOPort  Port=1  Side=Left
  in_b : PMIOPort  Port=2  Side=Left
  in_c : PMIOPort  Port=3  Side=Left
  out_a : PMIOPort  Port=4  Side=Right
  out_b : PMIOPort  Port=5  Side=Right
  out_c : PMIOPort  Port=6  Side=Right
  Vabc : Outport
  Iabc : Outport  Port=2
  wires:
  Close switch/1(Out1) -> Contactor/1(com)
  Memory/1 -> Close switch/1(In1)
  Complex to Real-Imag1/1 -> Iabc/1
  Complex to Real-Imag/1 -> Vabc/1
  P.O.R  and CTA/2 -> Complex to Real-Imag1/1
  P.O.R  and CTA/1 -> Complex to Real-Imag/1
  GLC/1 -> Memory/1
  connections:
  Contactor/RConn3 -- out_c/RConn1
  Contactor/RConn1 -- out_a/RConn1
  P.O.R  and CTA/RConn2 -- Contactor/LConn2
  Contactor/LConn3 -- P.O.R  and CTA/RConn3
  P.O.R  and CTA/LConn3 -- in_c/RConn1
  in_b/RConn1 -- P.O.R  and CTA/LConn2
  P.O.R  and CTA/LConn1 -- in_a/RConn1
  Contactor/LConn1 -- P.O.R  and CTA/RConn1
  out_b/RConn1 -- Contactor/RConn2

== system Generator_Lib/Integrated Drive/IDG ==
  Tur : Inport
  Constant : Constant  Value=12000*pi/30
  Terminator : Terminator
  rpm2 radps : Gain  Gain=pi/30
  Dr : Outport
  wires:
  rpm2 radps/1 -> Terminator/1
  Tur/1 -> rpm2 radps/1
  Constant/1 -> Dr/1

== system Generator_Lib/Integrated Drive/Sensing ==
  In1 : Inport
  Data : Subsystem
  Mux : Mux  Inputs=3
  tag scope: Gen1Data=global
  wires:
  Mux/1 -> [Gen1Data]
  In1/1 -> Data/1(B)
  Data/1(w) -> Mux/1
  Data/2(Vf) -> Mux/2
  Data/3(Pe) -> Mux/3

== system Generator_Lib/Integrated Drive/Vab ==
  Voltage Measurement : powerlib/Measurements/Voltage Measurement  PhasorSimulation=off  OutputType=Magnitude  PSBequivalent=0
  + : PMIOPort  Port=1  Side=Right
  - : PMIOPort  Port=2  Side=Right
  tag scope: Gen1_Vab=global
  wires:
  Voltage Measurement/1 -> [Gen1_Vab]
  connections:
  Voltage Measurement/LConn2 -- -/RConn1
  Voltage Measurement/LConn1 -- +/RConn1

== system Generator_Lib/VSCF Cycloconverter/AC Generator Cycloconverter ==
  rpm : Inport
  Cycloconverter control (Vsync) : Subsystem
  Ground1 : powerlib/Elements/Ground  LConnTagsString=a
  Ideal Source : Subsystem
  Load Measurements : powerlib/Measurements/Three-Phase V-I Measurement  VoltageMeasurement=phase-to-ground  SetLabelV=on  LabelV=Vload  Vpu=off  VpuLL=off  CurrentMeasurement=yes  SetLabelI=on  LabelI=Iload  Ipu=off  Pbase=100e6  Vbase=500e3  OutputType=Complex  PhasorSimulation=off  PSBequivalent=0
  Phase A Cycloconverter : Subsystem
  Phase B Cycloconverter : Subsystem
  Phase C Cycloconverter : Subsystem
  Source Measurements : powerlib/Measurements/Three-Phase V-I Measurement  VoltageMeasurement=phase-to-ground  SetLabelV=on  LabelV=Vsource  Vpu=off  VpuLL=off  CurrentMeasurement=yes  SetLabelI=on  LabelI=Isource  Ipu=off  Pbase=100e6  Vbase=500e3  OutputType=Complex  PhasorSimulation=off  PSBequivalent=0
  Three-Phase Transformer (Two Windings)1 : powerlib/Elements/Three-Phase Transformer (Two Windings)  Winding1Connection=Delta (D1)  UNITS=pu  NominalPower=[3e6 3000]  Winding1=[200 0 0]  Winding2Connection=Delta (D1)  Winding2=[200/sqrt(3) 1e-8 0]  SetSaturation=off  Rm=Inf  Lm=Inf  Saturation=[ 0,0 ; 0.0024,1.2 ; 1.0,1.52 ]  Hysteresis=off  DataFile='hysteresis'  SetInitialFlux=off  InitialFluxes=[ 0.8 , -0.8 , 0.7 ]  Measurements=None  MoreParameters=off  BreakLoop=off  DataType=off  TransfoNumber=1
  Three-Phase Transformer (Two Windings)2 : powerlib/Elements/Three-Phase Transformer (Two Windings)  Winding1Connection=Delta (D1)  UNITS=pu  NominalPower=[3e6 3000]  Winding1=[200 0 0]  Winding2Connection=Delta (D1)  Winding2=[200/sqrt(3) 1e-8 0]  SetSaturation=off  Rm=Inf  Lm=Inf  Saturation=[ 0,0 ; 0.0024,1.2 ; 1.0,1.52 ]  Hysteresis=off  DataFile='hysteresis'  SetInitialFlux=off  InitialFluxes=[ 0.8 , -0.8 , 0.7 ]  Measurements=None  MoreParameters=off  BreakLoop=off  DataType=off  TransfoNumber=1
  Three-Phase Transformer (Two Windings)3 : powerlib/Elements/Three-Phase Transformer (Two Windings)  Winding1Connection=Delta (D1)  UNITS=pu  NominalPower=[3e6 3000]  Winding1=[200 0 0]  Winding2Connection=Delta (D1)  Winding2=[200/sqrt(3) 1e-8 0]  SetSaturation=off  Rm=Inf  Lm=Inf  Saturation=[ 0,0 ; 0.0024,1.2 ; 1.0,1.52 ]  Hysteresis=off  DataFile='hysteresis'  SetInitialFlux=off  InitialFluxes=[ 0.8 , -0.8 , 0.7 ]  Measurements=None  MoreParameters=off  BreakLoop=off  DataType=off  TransfoNumber=1
  Vsync Measurement : powerlib/Measurements/Three-Phase V-I Measurement  VoltageMeasurement=phase-to-phase  SetLabelV=on  LabelV=Vsync  Vpu=off  VpuLL=off  CurrentMeasurement=no  SetLabelI=off  LabelI=Iabc  Ipu=off  Pbase=100e6  Vbase=500e3  OutputType=Complex  PhasorSimulation=off  PSBequivalent=0
  A : PMIOPort  Port=1  Side=Right
  B : PMIOPort  Port=2  Side=Right
  C : PMIOPort  Port=3  Side=Right
  wires:
  rpm/1 -> Ideal Source/1(rpm)
  connections:
  Load Measurements/RConn1 -- A/RConn1
  Phase A Cycloconverter/LConn2 -- Vsync Measurement/RConn2
  Three-Phase Transformer (Two Windings)3/RConn3 -- Vsync Measurement/LConn3
  Phase C Cycloconverter/RConn2 -- Phase A Cycloconverter/RConn2 -- Phase B Cycloconverter/RConn2 -- Ground1/LConn1
  Three-Phase Transformer (Two Windings)2/RConn2 -- Phase C Cycloconverter/LConn2
  Source Measurements/RConn3 -- Three-Phase Transformer (Two Windings)3/LConn3 -- Three-Phase Transformer (Two Windings)2/LConn3 -- Three-Phase Transformer (Two Windings)1/LConn3
  Phase B Cycloconverter/RConn1 -- Load Measurements/LConn2
  Vsync Measurement/RConn1 -- Phase A Cycloconverter/LConn1
  Phase B Cycloconverter/LConn1 -- Three-Phase Transformer (Two Windings)1/RConn1
  Phase B Cycloconverter/LConn2 -- Three-Phase Transformer (Two Windings)1/RConn2
  Three-Phase Transformer (Two Windings)3/RConn1 -- Vsync Measurement/LConn1
  Phase C Cycloconverter/LConn1 -- Three-Phase Transformer (Two Windings)2/RConn1
  Phase A Cycloconverter/RConn1 -- Load Measurements/LConn1
  Source Measurements/RConn1 -- Three-Phase Transformer (Two Windings)3/LConn1 -- Three-Phase Transformer (Two Windings)2/LConn1 -- Three-Phase Transformer (Two Windings)1/LConn1
  Source Measurements/RConn2 -- Three-Phase Transformer (Two Windings)3/LConn2 -- Three-Phase Transformer (Two Windings)2/LConn2 -- Three-Phase Transformer (Two Windings)1/LConn2
  Phase C Cycloconverter/RConn1 -- Load Measurements/LConn3
  Vsync Measurement/RConn3 -- Phase A Cycloconverter/LConn3
  Load Measurements/RConn3 -- C/RConn1
  Phase C Cycloconverter/LConn3 -- Three-Phase Transformer (Two Windings)2/RConn3
  Source Measurements/LConn2 -- Ideal Source/RConn2
  Three-Phase Transformer (Two Windings)3/RConn2 -- Vsync Measurement/LConn2
  Ideal Source/RConn1 -- Source Measurements/LConn1
  Load Measurements/RConn2 -- B/RConn1
  Ideal Source/RConn3 -- Source Measurements/LConn3
  Three-Phase Transformer (Two Windings)1/RConn3 -- Phase B Cycloconverter/LConn3

== system Generator_Lib/VSCF Cycloconverter/Generator Control Breaker (GCB) ==
  GLC : Inport
  Close switch : Subsystem
  Complex to Real-Imag : ComplexToRealImag  Output=Real
  Complex to Real-Imag1 : ComplexToRealImag  Output=Real
  Contactor : Subsystem
  Memory : Memory
  P.O.R  and CTA : powerlib/Measurements/Three-Phase V-I Measurement  VoltageMeasurement=phase-to-phase  SetLabelV=off  LabelV=Vabc_Gen1  Vpu=off  VpuLL=off  CurrentMeasurement=yes  SetLabelI=off  LabelI=Iabc_Gen1  Ipu=off  Pbase=100e6  Vbase=500e3  OutputType=Complex  PhasorSimulation=off  PSBequivalent=0
  in_a : PMIOPort  Port=1  Side=Left
  in_b : PMIOPort  Port=2  Side=Left
  in_c : PMIOPort  Port=3  Side=Left
  out_a : PMIOPort  Port=4  Side=Right
  out_b : PMIOPort  Port=5  Side=Right
  out_c : PMIOPort  Port=6  Side=Right
  Vabc : Outport
  Iabc : Outport  Port=2
  wires:
  Close switch/1(Out1) -> Contactor/1(com)
  Memory/1 -> Close switch/1(In1)
  Complex to Real-Imag1/1 -> Iabc/1
  Complex to Real-Imag/1 -> Vabc/1
  P.O.R  and CTA/2 -> Complex to Real-Imag1/1
  P.O.R  and CTA/1 -> Complex to Real-Imag/1
  GLC/1 -> Memory/1
  connections:
  Contactor/RConn3 -- out_c/RConn1
  Contactor/RConn1 -- out_a/RConn1
  P.O.R  and CTA/RConn2 -- Contactor/LConn2
  Contactor/LConn3 -- P.O.R  and CTA/RConn3
  P.O.R  and CTA/LConn3 -- in_c/RConn1
  in_b/RConn1 -- P.O.R  and CTA/LConn2
  P.O.R  and CTA/LConn1 -- in_a/RConn1
  Contactor/LConn1 -- P.O.R  and CTA/RConn1
  out_b/RConn1 -- Contactor/RConn2

== system Generator_Lib/VSCF Cycloconverter/Vab ==
  Voltage Measurement : powerlib/Measurements/Voltage Measurement  PhasorSimulation=off  OutputType=Magnitude  PSBequivalent=0
  + : PMIOPort  Port=1  Side=Right
  - : PMIOPort  Port=2  Side=Right
  tag scope: Gen1_Vab=global
  wires:
  Voltage Measurement/1 -> [Gen1_Vab]
  connections:
  Voltage Measurement/LConn2 -- -/RConn1
  Voltage Measurement/LConn1 -- +/RConn1

== system Generator_Lib/VSCF DC Link/DC Link Gen ==
  rpm : Inport
  Ideal : Generator_Lib/DC Gen/Ideal  SystemSampleTime=-1
  A : PMIOPort  Port=1  Side=Right
  B : PMIOPort  Port=2  Side=Right
  C : PMIOPort  Port=3  Side=Right
  wires:
  rpm/1 -> Ideal/1
  connections:
  Ideal/RConn1 -- A/RConn1
  Ideal/RConn2 -- B/RConn1
  Ideal/RConn3 -- C/RConn1

== system Generator_Lib/VSCF DC Link/LC Filter ==
  Capacitor : powerlib/Elements/Three-Phase Series RLC Load  LConnTagsString=A|B|C  Configuration=Y (grounded)  NominalVoltage=200  NominalFrequency=400  ActivePower=0  InductivePower=0  CapacitivePower=3e3  Measurements=None  LoadType=constant Z
  Inductor : powerlib/Elements/Three-Phase Series RLC Branch  LConnTagsString=A|B|C  RConnTagsString=A|B|C  BranchType=L  Resistance=0  Inductance=2e-3*0.43  Capacitance=inf  Measurements=None
  A : PMIOPort  Port=1  Side=Left
  B : PMIOPort  Port=2  Side=Left
  C : PMIOPort  Port=3  Side=Left
  "A " : PMIOPort  Port=4  Side=Right
  "B " : PMIOPort  Port=5  Side=Right
  "C " : PMIOPort  Port=6  Side=Right
  connections:
  B/RConn1 -- Inductor/LConn2
  A/RConn1 -- Inductor/LConn1
  C/RConn1 -- Inductor/LConn3
  Inductor/RConn1 -- "A "/RConn1 -- Capacitor/LConn1
  Inductor/RConn2 -- "B "/RConn1 -- Capacitor/LConn2
  Inductor/RConn3 -- Capacitor/LConn3 -- "C "/RConn1

== system Generator_Lib/VSCF DC Link/Rect and Inv ==
  g : Inport
  C1 : powerlib/Elements/Parallel RLC Branch  LConnTagsString=a  RConnTagsString=__new0  BranchType=C  Resistance=inf  Inductance=inf  SetiL0=off  InitialCurrent=0  Capacitance=5000e-06  Setx0=on  InitialVoltage=797  Measurements=None
  L1 : powerlib/Elements/Series RLC Branch  LConnTagsString=__new0  RConnTagsString=__new0  BranchType=L  Resistance=1.0  Inductance=200e-6  SetiL0=off  InitialCurrent=0  Capacitance=1.0  Setx0=off  InitialVoltage=0  Measurements=None
  PWM IGBT Inverter : powerlib/Power Electronics/Universal Bridge  Arms=3  SnubberResistance=5000  SnubberCapacitance=inf  Device=IGBT / Diodes  Ron=1e-3  Lon=0  ForwardVoltages="[  0.0  0.0  ]"  ForwardVoltage=.8  GTOparameters=[ 1e-6 ,1e-6 ]  IGBTparameters=[ 1e-6 , 2e-6 ]  Measurements=Device currents  Measurements_2=None  converterType=Rectifier
  Rectifier : powerlib/Power Electronics/Universal Bridge  Arms=3  SnubberResistance=100  SnubberCapacitance=0.1e-6  Device=Diodes  Ron=1e-3  Lon=0  ForwardVoltages="[  0.8  0.8  ]"  ForwardVoltage=.8  GTOparameters=[ 10e-6 , 20e-6 ]  IGBTparameters=[ 1e-6 , 2e-6 ]  Measurements=Device currents  Measurements_2=None  converterType=Rectifier
  Subsystem3 : Subsystem
      mask Display: disp('S')
  Ar : PMIOPort  Port=1  Side=Left
  Ai : PMIOPort  Port=2  Side=Right
  Br : PMIOPort  Port=3  Side=Left
  Bi : PMIOPort  Port=4  Side=Right
  Cr : PMIOPort  Port=5  Side=Left
  Ci : PMIOPort  Port=6  Side=Right
  wires:
  g/1 -> PWM IGBT Inverter/1
  connections:
  PWM IGBT Inverter/LConn3 -- Ci/RConn1
  Rectifier/RConn1 -- L1/LConn1
  PWM IGBT Inverter/RConn2 -- C1/RConn1 -- Rectifier/RConn2 -- Subsystem3/RConn1
  L1/RConn1 -- C1/LConn1 -- PWM IGBT Inverter/RConn1 -- Subsystem3/LConn1
  Cr/RConn1 -- Rectifier/LConn3
  Ar/RConn1 -- Rectifier/LConn1
  Rectifier/LConn2 -- Br/RConn1
  PWM IGBT Inverter/LConn2 -- Bi/RConn1
  PWM IGBT Inverter/LConn1 -- Ai/RConn1

== system Generator_Lib/VSCF DC Link/Regulator ==
  Vref (pu) : Inport
  Vabc (pu) : Inport  Port=2
  Discrete PWM Generator : powerlib_extras/Discrete  Control Blocks/Discrete PWM Generator  GeneratorMode="3-arm  bridge (6 pulses)"  Fc=10000  Ts=Ts  Internal=off  mIndex=0.4  Freq=60  Phase=0
  Unit Delay1 : UnitDelay  SampleTime=Ts
  Voltage Regulator : Subsystem  mask(Voltage Regulator){Kp=0.4, Ki=500, Ts=Ts}
      mask prompts: Kp "Proportional gain  Kp:"; Ki "Integral gain Ki:"; Ts "Sample time (s) :"
  g : Outport
  wires:
  Voltage Regulator/1(Vabc_inv) -> Discrete PWM Generator/1
  Vabc (pu)/1 -> Voltage Regulator/2(Vabc (pu))
  Vref (pu)/1 -> Voltage Regulator/1(Vd_ref (pu))
  Discrete PWM Generator/1 -> Unit Delay1/1
  Unit Delay1/1 -> g/1

== system Generator_Lib/VSCF DC Link/Subsystem2 ==
  Ground : powerlib/Elements/Ground  LConnTagsString=a
  Vdc1 : powerlib/Measurements/Voltage Measurement  Tag=PoWeRsYsTeMmEaSuReMeNt  PhasorSimulation=off  OutputType=Magnitude  PSBequivalent=0
  Conn1 : PMIOPort  Port=1  Side=Left
  tag scope: Va_Src=global
  wires:
  Vdc1/1 -> [Va_Src]
  connections:
  Vdc1/LConn1 -- Conn1/RConn1
  Ground/LConn1 -- Vdc1/LConn2

== system Generator_Lib/VSCF DC Link/Subsystem4 ==
  Ground : powerlib/Elements/Ground  LConnTagsString=a
  Vdc1 : powerlib/Measurements/Voltage Measurement  Tag=PoWeRsYsTeMmEaSuReMeNt  PhasorSimulation=off  OutputType=Magnitude  PSBequivalent=0
  Conn1 : PMIOPort  Port=1  Side=Left
  tag scope: Va_Load=global
  wires:
  Vdc1/1 -> [Va_Load]
  connections:
  Ground/LConn1 -- Vdc1/LConn2
  Vdc1/LConn1 -- Conn1/RConn1

== system Generator_Lib/VSCF DC Link/Subsystem5 ==
  Vdc : powerlib/Measurements/Voltage Measurement  Tag=PoWeRsYsTeMmEaSuReMeNt  PhasorSimulation=off  OutputType=Magnitude  PSBequivalent=0
  + : PMIOPort  Port=1  Side=Left
  - : PMIOPort  Port=2  Side=Left
  tag scope: Vab_Inv=global
  wires:
  Vdc/1 -> [Vab_Inv]  "Vdc"
  connections:
  -/RConn1 -- Vdc/LConn2
  Vdc/LConn1 -- +/RConn1

== system Generator_Lib/Cyclo Gen/Ideal/Cycloconverter control (Vsync) ==
  Cyclo Firing Control PhA : Subsystem
  Cyclo Firing Control PhB : Subsystem
  Cyclo Firing Control PhC : Subsystem
  Demux : Demux  Outputs=3
  Discrete-Time Integrator : DiscreteIntegrator  SampleTime=Ts  ICPrevOutput=DiscIntNeverNeededParam  ICPrevScaledInput=DiscIntNeverNeededParam
  Gain1 : Gain  Gain=2*pi
  Gain2 : Gain  Gain=1/(200*sqrt(2/3))
  Gain5 : Gain  Gain=200*sqrt(2/3)
  Sine : Subsystem
  output frequency (Hz) : simulink/Sources/Repeating Sequence  rep_seq_t=[0 10]  rep_seq_y=[1 1]*400
  output voltage (V peak) : simulink/Sources/Repeating Sequence  rep_seq_t=[0 10]  rep_seq_y=[1 1]*200*sqrt(2/3)
  tag scope: Ea=global, vab=global, vbc=global, vca=global
  wires:
  Discrete-Time Integrator/1 -> Sine/2(theta)
  Sine/2(b) -> Cyclo Firing Control PhB/1(Eref)
  Sine/1(a) -> Cyclo Firing Control PhA/1(Eref), Gain5/1
  Sine/3(c) -> Cyclo Firing Control PhC/1(Eref)
  output frequency (Hz)/1 -> Gain1/1
  Gain1/1 -> Discrete-Time Integrator/1
  Gain5/1 -> [Ea]
  output voltage (V peak)/1 -> Gain2/1
  Gain2/1 -> Sine/1(Eref)
  [Vsync] -> Demux/1
  Demux/1 -> [vab]
  Demux/2 -> [vbc]
  Demux/3 -> [vca]
  [input_freq] -> Cyclo Firing Control PhC/2(freq (Hz)), Cyclo Firing Control PhA/2(freq (Hz)), Cyclo Firing Control PhB/2(freq (Hz))

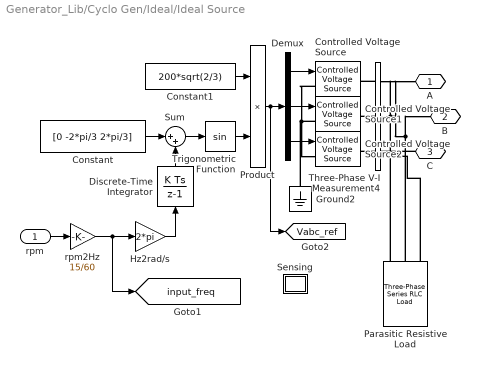
== system Generator_Lib/Cyclo Gen/Ideal/Ideal Source ==
  rpm : Inport
  Constant : Constant  Value=[0 -2*pi/3 2*pi/3]
  Constant1 : Constant  Value=200*sqrt(2/3)
  Controlled Voltage Source : powerlib/Electrical Sources/Controlled Voltage Source  Initialize=off  Source_Type=AC  Amplitude=0  Phase=0  Frequency=0  Measurements=None
  Controlled Voltage Source1 : powerlib/Electrical Sources/Controlled Voltage Source  Initialize=off  Source_Type=AC  Amplitude=0  Phase=0  Frequency=0  Measurements=None
  Controlled Voltage Source2 : powerlib/Electrical Sources/Controlled Voltage Source  Initialize=off  Source_Type=AC  Amplitude=0  Phase=0  Frequency=0  Measurements=None
  Demux : Demux  Outputs=3
  Discrete-Time Integrator : DiscreteIntegrator  SampleTime=Ts  ICPrevOutput=DiscIntNeverNeededParam  ICPrevScaledInput=DiscIntNeverNeededParam
  Ground2 : powerlib/Elements/Ground  LConnTagsString=a
  Hz2rad/s : Gain  Gain=2*pi
  Parasitic Resistive Load : powerlib/Elements/Three-Phase Series RLC Load  LConnTagsString=A|B|C  Configuration=Y (grounded)  NominalVoltage=200  NominalFrequency=400  ActivePower=5000  InductivePower=0  CapacitivePower=0  Measurements=None  LoadType=constant Z
  Product : Product
  Sensing : Subsystem
      mask Display: disp('S')
  Sum : Sum  Inputs=|++
  Three-Phase V-I Measurement4 : powerlib/Measurements/Three-Phase V-I Measurement  VoltageMeasurement=phase-to-ground  SetLabelV=on  LabelV=Vabc_Gen1Only  Vpu=off  VpuLL=off  CurrentMeasurement=yes  SetLabelI=on  LabelI=Iabc_Gen1Only  Ipu=off  Pbase=100e6  Vbase=500e3  OutputType=Magnitude  PhasorSimulation=on  PSBequivalent=0
  Trigonometric Function : Trigonometry
  rpm2Hz : Gain  Gain=15/60
  A : PMIOPort  Port=1  Side=Right
  B : PMIOPort  Port=2  Side=Right
  C : PMIOPort  Port=3  Side=Right
  tag scope: Vabc_ref=global, input_freq=global
  wires:
  rpm/1 -> rpm2Hz/1
  Discrete-Time Integrator/1 -> Sum/2
  Constant1/1 -> Product/1
  Constant/1 -> Sum/1
  Hz2rad/s/1 -> Discrete-Time Integrator/1
  Sum/1 -> Trigonometric Function/1
  Trigonometric Function/1 -> Product/2
  Product/1 -> [Vabc_ref], Demux/1
  Demux/1 -> Controlled Voltage Source/1
  Demux/2 -> Controlled Voltage Source1/1
  Demux/3 -> Controlled Voltage Source2/1
  rpm2Hz/1 -> [input_freq], Hz2rad/s/1
  connections:
  Controlled Voltage Source/LConn1 -- Ground2/LConn1 -- Controlled Voltage Source2/LConn1 -- Controlled Voltage Source1/LConn1
  Three-Phase V-I Measurement4/LConn2 -- Controlled Voltage Source1/RConn1
  Three-Phase V-I Measurement4/LConn1 -- Controlled Voltage Source/RConn1
  Three-Phase V-I Measurement4/LConn3 -- Controlled Voltage Source2/RConn1
  C/RConn1 -- Parasitic Resistive Load/LConn3 -- Three-Phase V-I Measurement4/RConn3
  Three-Phase V-I Measurement4/RConn2 -- B/RConn1 -- Parasitic Resistive Load/LConn2
  Three-Phase V-I Measurement4/RConn1 -- A/RConn1 -- Parasitic Resistive Load/LConn1

== system Generator_Lib/Cyclo Gen/Ideal/Phase A Cycloconverter ==
  negative cycle : powerlib/Power Electronics/Universal Bridge  Arms=3  SnubberResistance=1e3  SnubberCapacitance=1e-7  Device=Thyristors  Ron=1e-5  Lon=0  ForwardVoltages="[  0  0  ]"  ForwardVoltage=0  GTOparameters=[ 10e-6 , 20e-6 ]  IGBTparameters=[ 1e-6 , 2e-6 ]  Measurements=None  Measurements_2=None  converterType=Rectifier
  positive cycle : powerlib/Power Electronics/Universal Bridge  Arms=3  SnubberResistance=1e3  SnubberCapacitance=1e-7  Device=Thyristors  Ron=1e-5  Lon=0  ForwardVoltages="[  0  0  ]"  ForwardVoltage=0  GTOparameters=[ 10e-6 , 20e-6 ]  IGBTparameters=[ 1e-6 , 2e-6 ]  Measurements=None  Measurements_2=None  converterType=Rectifier
  VA+ : PMIOPort  Tag=PMCPort  Port=1  Side=Right
  VA- : PMIOPort  Tag=PMCPort  Port=2  Side=Right
  A : PMIOPort  Tag=PMCPort  Port=3  Side=Left
  B : PMIOPort  Tag=PMCPort  Port=4  Side=Left
  C : PMIOPort  Tag=PMCPort  Port=5  Side=Left
  wires:
  [PhAgp] -> positive cycle/1
  [PhAgn] -> negative cycle/1
  connections:
  A/RConn1 -- positive cycle/LConn1 -- negative cycle/LConn1
  B/RConn1 -- positive cycle/LConn2 -- negative cycle/LConn2
  C/RConn1 -- positive cycle/LConn3 -- negative cycle/LConn3
  negative cycle/RConn1 -- positive cycle/RConn2 -- VA-/RConn1
  positive cycle/RConn1 -- VA+/RConn1 -- negative cycle/RConn2

== system Generator_Lib/Cyclo Gen/Ideal/Phase B Cycloconverter ==
  negative cycle : powerlib/Power Electronics/Universal Bridge  Arms=3  SnubberResistance=1e3  SnubberCapacitance=1e-7  Device=Thyristors  Ron=1e-5  Lon=0  ForwardVoltages="[  0  0  ]"  ForwardVoltage=0  GTOparameters=[ 10e-6 , 20e-6 ]  IGBTparameters=[ 1e-6 , 2e-6 ]  Measurements=None  Measurements_2=None  converterType=Rectifier
  positive cycle : powerlib/Power Electronics/Universal Bridge  Arms=3  SnubberResistance=1e3  SnubberCapacitance=1e-7  Device=Thyristors  Ron=1e-5  Lon=0  ForwardVoltages="[  0  0  ]"  ForwardVoltage=0  GTOparameters=[ 10e-6 , 20e-6 ]  IGBTparameters=[ 1e-6 , 2e-6 ]  Measurements=None  Measurements_2=None  converterType=Rectifier
  VB+ : PMIOPort  Tag=PMCPort  Port=1  Side=Right
  VB- : PMIOPort  Tag=PMCPort  Port=2  Side=Right
  A : PMIOPort  Tag=PMCPort  Port=3  Side=Left
  B : PMIOPort  Tag=PMCPort  Port=4  Side=Left
  C : PMIOPort  Tag=PMCPort  Port=5  Side=Left
  wires:
  [PhBgn] -> negative cycle/1
  [PhBgp] -> positive cycle/1
  connections:
  negative cycle/RConn2 -- VB+/RConn1 -- positive cycle/RConn1
  VB-/RConn1 -- positive cycle/RConn2 -- negative cycle/RConn1
  negative cycle/LConn3 -- positive cycle/LConn3 -- C/RConn1
  negative cycle/LConn2 -- B/RConn1 -- positive cycle/LConn2
  negative cycle/LConn1 -- positive cycle/LConn1 -- A/RConn1
